simulink model "MLIB_Round_BAM_F32"  (Simulink 7.3)
settings: Solver=ode45  StartTime=0.0  StopTime=10.0  RelTol=1e-3
settings Model: Creator=B17364  LastModifiedBy=B17364

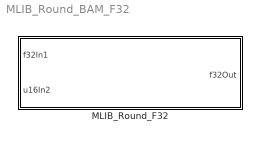
== system MLIB_Round_BAM_F32 ==
  MLIB_Round_F32 : Subsystem  mask(MLIB_Round_F32){}
      mask help: Bit accurate model of the fuction rounds the first input value for number of digits defined by second parameter and saturate automaticaly. All parameters as well as input and output are 32bit integers.
      mask init:
      | pos = get_param(gcb, 'Position');width = pos(3) - pos(1); height = pos(4) - pos(2);tX=width/2;tY=height*0.9;
      mask Display: color('black');port_label('input',1,'f32In1');port_label('input',2,'u16In2');port_label('output',1,'f32Out');color('black');disp('MLIB_Round_F32');color('blue');text(tX,tY, 'BAM', 'horizontalAlignment', 'center');

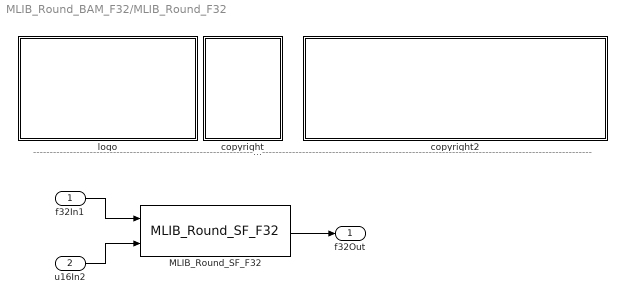
== system MLIB_Round_BAM_F32/MLIB_Round_F32 ==
  note: ---------------------------------------------------------------------------------------------------------------------------------------------------------------------------------------------------
  f32In1 : Inport  OutDataType=fixdt(1, 16)  OutScaling=2^0
  u16In2 : Inport  Port=2  OutDataType=fixdt(1, 16)  OutScaling=2^0
  MLIB_Round_SF_F32 : S-Function  FunctionName=MLIB_Round_SF_F32  EnableBusSupport=off
  copyright : Subsystem
      mask Display: text(10,90,'FILE:');text(10,75,'DESRIPTION:')text(10,60,'COPYRIGHT:')text(10,45,'VERSION:')text(10,30,'DATE:')
  copyright2 : Subsystem
      mask Display: text(10,90,'MLIB_Round_BAM_F32.mdl');text(10,75,'Round the first input value.');text(10,60,'Freescale')text(10,45,'0.1');text(10,30,'02-Sep-2011');
  logo : Subsystem
      mask Display: image(imread('logo.jpg'))
  f32Out : Outport  OutDataType=fixdt(1, 16)  OutScaling=2^0
  wires:
  f32In1/1 -> MLIB_Round_SF_F32/1
  u16In2/1 -> MLIB_Round_SF_F32/2
  MLIB_Round_SF_F32/1 -> f32Out/1

== system MLIB_Round_BAM_F32/MLIB_Round_F32/copyright ==

== system MLIB_Round_BAM_F32/MLIB_Round_F32/copyright2 ==

== system MLIB_Round_BAM_F32/MLIB_Round_F32/logo ==
